simulink model "Delivery"  (R2023a)
settings: Solver=ode1  StartTime=0.0  StopTime=T_stop  FixedStep=Ts  MaxStep=0.001  RelTol=1e-3  AbsTol=1e-3
PreLoadFcn:
  | Quadcopter_EMech_param_Ex1
model workspace (MATLAB code in the model file):
  | load('xy_data_membrane.mat');
undefined symbols (not defined in the file): initialAltitude, Jm, kd_altitude, kd_attitude, ki_altitude, ki_attitude, kp_altitude, kp_attitude, m_total, p, planedepth, planex, planey, psim, targetX, targetY, timespot, Tmax, Vdc, X, x0, xrot, Y, y0, yrot, Z, zrot
libraries: sm_lib x98, nesl_utility x69, fl_lib x60, ee_lib x12, slpidlib x4, Library_Ex1 x2
(part 7 of 7)

== system Delivery/Quadcopter/propeller4/Sensing w a1/Hall sensor ==
  theta : Inport
  Constant : Constant  Value=-60
  Constant1 : Constant  Value=120
  Constant2 : Constant  Value=60
  Constant3 : Constant  Value=-120
  Constant4 : Constant  Value=-180
  Constant5 : Constant  Value=0
  Logical Operator : Logic  AllPortsSameDT=off  OutDataTypeStr=boolean
  Logical Operator1 : Logic  Operator=OR  AllPortsSameDT=off  OutDataTypeStr=boolean
  Logical Operator2 : Logic  AllPortsSameDT=off  OutDataTypeStr=boolean
  Mux : Mux  Inputs=3
  Relational Operator1 : RelationalOperator  Operator=<=
  Relational Operator2 : RelationalOperator
  Relational Operator3 : RelationalOperator  Operator=<=
  Relational Operator4 : RelationalOperator
  Relational Operator5 : RelationalOperator  Operator=<=
  Relational Operator6 : RelationalOperator
  Subsystem : Subsystem
  Hall : Outport  VectorParamsAs1DForOutWhenUnconnected=off
  wires:
  Constant3/1 -> Relational Operator3/2
  Logical Operator2/1 -> Mux/3
  Logical Operator1/1 -> Mux/2
  Logical Operator/1 -> Mux/1
  Relational Operator5/1 -> Logical Operator2/2
  Relational Operator6/1 -> Logical Operator2/1
  Constant4/1 -> Relational Operator6/2
  Constant5/1 -> Relational Operator5/2
  Relational Operator3/1 -> Logical Operator1/2
  Mux/1 -> Hall/1
  Relational Operator2/1 -> Logical Operator/1
  Relational Operator1/1 -> Logical Operator/2
  Subsystem/1(deg) -> Relational Operator4/1, Relational Operator3/1, Relational Operator5/1, Relational Operator6/1, Relational Operator1/1, Relational Operator2/1
  Constant/1 -> Relational Operator2/2
  Relational Operator4/1 -> Logical Operator1/1
  Constant1/1 -> Relational Operator1/2
  Constant2/1 -> Relational Operator4/2
  theta/1 -> Subsystem/1(theta)

== system Delivery/Quadcopter/propeller1/Commutation/Commutation/Bit concatenate ==
  u : Inport
  Gain : Gain  Gain=[4 2 1]  Multiplication=Matrix(K*u)
  Sum of Elements : Sum  Inputs=+
  y : Outport  VectorParamsAs1DForOutWhenUnconnected=off
  wires:
  u/1 -> Gain/1
  Gain/1 -> Sum of Elements/1
  Sum of Elements/1 -> y/1

== system Delivery/Quadcopter/propeller1/Sensing w a1/Hall sensor/Subsystem ==
  theta : Inport
  Trigonometric Function : Trigonometry  Operator=sincos
  Trigonometric Function2 : Trigonometry  Operator=atan2
  mech->elec : Gain  Gain=p
  rad->deg : Gain  Gain=180/pi  SaturateOnIntegerOverflow=on  OutDataTypeStr=Inherit: Same as input  ParamDataTypeStr=Inherit: Same as input
  deg : Outport  VectorParamsAs1DForOutWhenUnconnected=off
  wires:
  Trigonometric Function2/1 -> rad->deg/1
  Trigonometric Function/1 -> Trigonometric Function2/1
  theta/1 -> mech->elec/1
  rad->deg/1 -> deg/1
  Trigonometric Function/2 -> Trigonometric Function2/2
  mech->elec/1 -> Trigonometric Function/1

== system Delivery/Quadcopter/propeller2/Commutation/Commutation/Bit concatenate ==
  u : Inport
  Gain : Gain  Gain=[4 2 1]  Multiplication=Matrix(K*u)
  Sum of Elements : Sum  Inputs=+
  y : Outport  VectorParamsAs1DForOutWhenUnconnected=off
  wires:
  u/1 -> Gain/1
  Gain/1 -> Sum of Elements/1
  Sum of Elements/1 -> y/1

== system Delivery/Quadcopter/propeller2/Sensing w a1/Hall sensor/Subsystem ==
  theta : Inport
  Trigonometric Function : Trigonometry  Operator=sincos
  Trigonometric Function2 : Trigonometry  Operator=atan2
  mech->elec : Gain  Gain=p
  rad->deg : Gain  Gain=180/pi  SaturateOnIntegerOverflow=on  OutDataTypeStr=Inherit: Same as input  ParamDataTypeStr=Inherit: Same as input
  deg : Outport  VectorParamsAs1DForOutWhenUnconnected=off
  wires:
  Trigonometric Function2/1 -> rad->deg/1
  Trigonometric Function/1 -> Trigonometric Function2/1
  theta/1 -> mech->elec/1
  rad->deg/1 -> deg/1
  Trigonometric Function/2 -> Trigonometric Function2/2
  mech->elec/1 -> Trigonometric Function/1

== system Delivery/Quadcopter/propeller3 /Commutation/Commutation/Bit concatenate ==
  u : Inport
  Gain : Gain  Gain=[4 2 1]  Multiplication=Matrix(K*u)
  Sum of Elements : Sum  Inputs=+
  y : Outport  VectorParamsAs1DForOutWhenUnconnected=off
  wires:
  u/1 -> Gain/1
  Gain/1 -> Sum of Elements/1
  Sum of Elements/1 -> y/1

== system Delivery/Quadcopter/propeller3 /Sensing w a1/Hall sensor/Subsystem ==
  theta : Inport
  Trigonometric Function : Trigonometry  Operator=sincos
  Trigonometric Function2 : Trigonometry  Operator=atan2
  mech->elec : Gain  Gain=p
  rad->deg : Gain  Gain=180/pi  SaturateOnIntegerOverflow=on  OutDataTypeStr=Inherit: Same as input  ParamDataTypeStr=Inherit: Same as input
  deg : Outport  VectorParamsAs1DForOutWhenUnconnected=off
  wires:
  Trigonometric Function2/1 -> rad->deg/1
  Trigonometric Function/1 -> Trigonometric Function2/1
  theta/1 -> mech->elec/1
  rad->deg/1 -> deg/1
  Trigonometric Function/2 -> Trigonometric Function2/2
  mech->elec/1 -> Trigonometric Function/1

== system Delivery/Quadcopter/propeller4/Commutation/Commutation/Bit concatenate ==
  u : Inport
  Gain : Gain  Gain=[4 2 1]  Multiplication=Matrix(K*u)
  Sum of Elements : Sum  Inputs=+
  y : Outport  VectorParamsAs1DForOutWhenUnconnected=off
  wires:
  u/1 -> Gain/1
  Gain/1 -> Sum of Elements/1
  Sum of Elements/1 -> y/1

== system Delivery/Quadcopter/propeller4/Sensing w a1/Hall sensor/Subsystem ==
  theta : Inport
  Trigonometric Function : Trigonometry  Operator=sincos
  Trigonometric Function2 : Trigonometry  Operator=atan2
  mech->elec : Gain  Gain=p
  rad->deg : Gain  Gain=180/pi  SaturateOnIntegerOverflow=on  OutDataTypeStr=Inherit: Same as input  ParamDataTypeStr=Inherit: Same as input
  deg : Outport  VectorParamsAs1DForOutWhenUnconnected=off
  wires:
  Trigonometric Function2/1 -> rad->deg/1
  Trigonometric Function/1 -> Trigonometric Function2/1
  theta/1 -> mech->elec/1
  rad->deg/1 -> deg/1
  Trigonometric Function/2 -> Trigonometric Function2/2
  mech->elec/1 -> Trigonometric Function/1

== matlab function Delivery/Manuver Controller/Attitude Controller/attitude planner ==
  data: des_pos input; des_vel input; des_yaw input; pos input; vel input; pitch_des output; roll_des output; yaw_des output; attitude input; T_drop input; t input; m_quad input; m_package input
function [pitch_des,roll_des,yaw_des] = attitude_planner(des_pos,des_vel,des_yaw,pos,vel,attitude, T_drop,t, m_quad, m_package)

%PID parameter value
% kp = 0.08^(3/2);
% kd = 0.53^(3/2);
kp = 0.199^(3/2);
kd = 0.849585^(3/2);

phi = attitude(1);
theta = attitude(2);
psi = attitude(3);


if T_drop == 0
    m_eff = m_quad + m_package;
else
    m_eff = m_quad;
end

% obtain the desired state
R_BI = [cos(theta)*cos(psi)                                    cos(theta)*sin(psi)                          -sin(theta);
    -cos(phi)*sin(psi)+sin(phi)*sin(theta)*cos(psi) cos(phi)*cos(psi)+sin(phi)*sin(theta)*sin(psi) sin(phi)*cos(theta);
    sin(phi)*sin(psi)+cos(phi)*sin(theta)*cos(psi) -sin(phi)*cos(psi)+cos(phi)*sin(theta)*sin(psi) cos(phi)*cos(theta)];

v_des = R_BI*((des_vel - vel) + kp*(des_pos - pos));

pitch_des   = (1/(9.81))*(kd*v_des(1)); 
roll_des   = (-1/(9.81))*(kd*v_des(2)); 
yaw_des = des_yaw;
end

== matlab function Delivery/Quadcopter/quad_body/Rot to Eul ==
  data: u input; theta_x output; theta_y output; theta_z output
function [theta_x,theta_y,theta_z] = fcn(u)

 theta = rotm2eul(u,'XYZ');
 theta_x = rad2deg(theta(1));
 theta_y = rad2deg(theta(2));
 theta_z = rad2deg(theta(3));
 
 
end

== matlab function Delivery/Manuver Controller/Waypoints Conversion ==
  data: way input; points1 output
function points1 = conversion(way)

counter_row=1;
counter_column=1;
points = zeros((length(way))/3,3);
for i = 1: length(way)
    if mod(i,3) == 0
        points(counter_row,counter_column) = way(i);
        counter_column = 1;
        counter_row = counter_row+1;
    else
        points(counter_row,counter_column) = way(i);
        counter_column = counter_column+1;
    end
end
tmp = points';
points1 = tmp;
end

== matlab function Delivery/Manuver Controller/Waypoint Trajectory Generator ==
  settings: updateMethod=DISCRETE
  data: t input; des_pos output; des_vel output; des_yaw output; homePose input; launch input; timespot input; waypoints input
function [des_pos,des_vel,des_yaw]  = traj_generator(t,homePose,launch,timespot,waypoints)
% This is the function used to calculate the trajectory for the given
% waypoints. The output of the function would be the desired state of 
% quadcopter, which includes the target position and velocity.
% This function should be used in sequence with attitude planner to give 
% desired pitch, roll and yaw angle of quadcopter.

persistent traj_startTime;

if launch == 1 && isempty(traj_startTime)
    traj_startTime = t;
    [des_pos, des_vel] = quinticpolytraj([homePose,waypoints], timespot, t-traj_startTime);
elseif launch == 1 && ~isempty(traj_startTime)
    [des_pos, des_vel] = quinticpolytraj([homePose,waypoints], timespot, t-traj_startTime);
else
    des_pos = homePose;
    des_vel = [0;0;0];
end
des_yaw = 0;
end
